simulink model "reduced_orig"  (R2018a)
settings: Solver=VariableStepAuto  StartTime=0.0  StopTime=10.0  RelTol=1e-3
undefined symbols (not defined in the file or in its folder): DiscIntNeverNeededParam
libraries: simulink x24
settings Model: Creator=ishaf  LastModifiedBy=ishaf

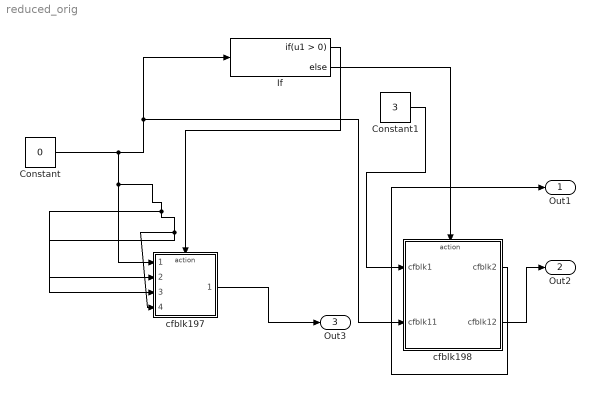
== system reduced_orig ==
  Constant : Constant  Value=0
  Constant1 : Constant  Value=3
  If : If
  cfblk197 : Subsystem  TreatAsAtomicUnit=on
  cfblk198 : Subsystem  TreatAsAtomicUnit=on
  Out1 : Outport
  Out2 : Outport  Port=2
  Out3 : Outport  Port=3
  wires:
  If/2 -> cfblk198/Action
  cfblk198/1(cfblk2) -> Out1/1
  If/1 -> cfblk197/Action
  cfblk198/2(cfblk12) -> Out2/1
  cfblk197/1(cfblk2) -> Out3/1
  Constant/1 -> cfblk197/1(cfblk1), cfblk197/2(cfblk14), cfblk197/4(cfblk16), cfblk197/3(cfblk15), cfblk198/2(cfblk11), If/1
  Constant1/1 -> cfblk198/1(cfblk1)

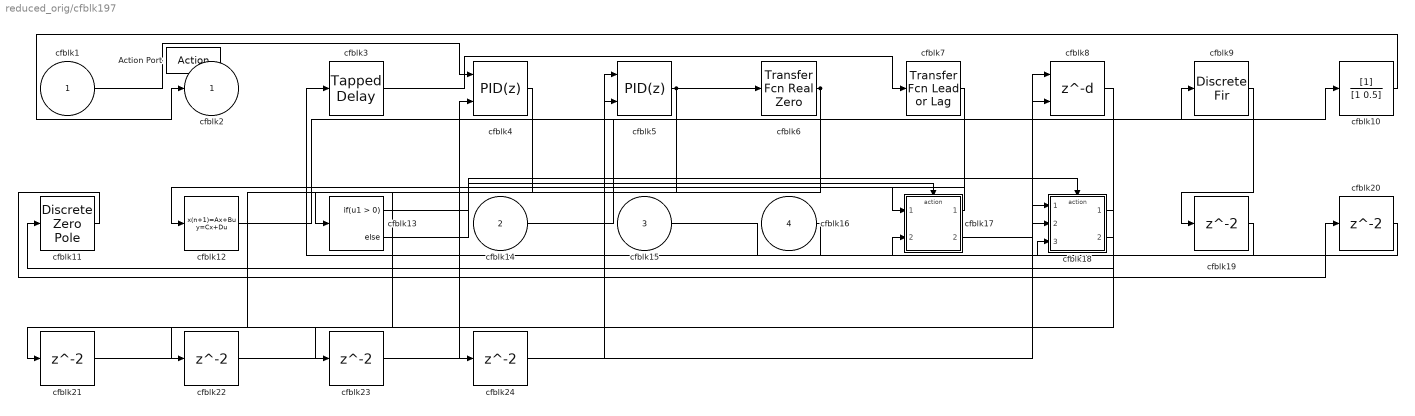
== system reduced_orig/cfblk197 ==
  cfblk1 : Inport
  cfblk14 : Inport  Port=2
  cfblk15 : Inport  Port=3
  cfblk16 : Inport  Port=4
  Action Port : ActionPort  ActionType=then
  cfblk10 : DiscreteFilter
  cfblk11 : DiscreteZeroPole  Poles=[0 0.5]  Gain=1  SampleTime=-1
  cfblk12 : DiscreteStateSpace  SampleTime=-1
  cfblk13 : If  SampleTime=1
  cfblk17 : Subsystem  TreatAsAtomicUnit=on
  cfblk18 : Subsystem  TreatAsAtomicUnit=on
  cfblk{19..24} (6 alike) : Delay
  cfblk3 : simulink/Discrete/Tapped Delay  vinit=0.0  samptime=-1  NumDelays=1  DelayOrder=Oldest  includeCurrent=off
  cfblk4 : simulink/Continuous/PID Controller (2DOF)  Controller=PID  TimeDomain=Discrete-time  SampleTime=-1  IntegratorMethod=Forward Euler  FilterMethod=Forward Euler  Form=Parallel  UseFilter=on  ControllerParametersSource=internal  P=1  I=1  D=0  N=100  b=1  c=1  InitialConditionSource=internal  InitialConditionForIntegrator=0  InitialConditionForFilter=0  ExternalReset=none  LimitOutput=off  UpperSaturationLimit=inf  LowerSaturationLimit=-inf  LinearizeAsGain=off  AntiWindupMode=none  Kb=1  TrackingMode=off  Kt=1  PParamMin=[]  PParamMax=[]  IParamMin=[]  IParamMax=[]  DParamMin=[]  DParamMax=[]  NParamMin=[]  NParamMax=[]  bParamMin=[]  bParamMax=[]  cParamMin=[]  cParamMax=[]  KbParamMin=[]  KbParamMax=[]  KtParamMin=[]  KtParamMax=[]  POutMin=[]  POutMax=[]  IOutMin=[]  IOutMax=[]  DOutMin=[]  DOutMax=[]  NOutMin=[]  NOutMax=[]  bOutMin=[]  bOutMax=[]  cOutMin=[]  cOutMax=[]  KbOutMin=[]  KbOutMax=[]  KtOutMin=[]  KtOutMax=[]  IntegratorOutMin=[]  IntegratorOutMax=[]  FilterOutMin=[]  FilterOutMax=[]  SumOutMin=[]  SumOutMax=[]  Sum1OutMin=[]  Sum1OutMax=[]  Sum2OutMin=[]  Sum2OutMax=[]  Sum3OutMin=[]  Sum3OutMax=[]  SumI1OutMin=[]  SumI1OutMax=[]  SumI2OutMin=[]  SumI2OutMax=[]  SumI3OutMin=[]  SumI3OutMax=[]  SumDOutMin=[]  SumDOutMax=[]  SaturationOutMin=[]  SaturationOutMax=[]  IntegratorContinuousStateAttributes=''  IntegratorStateMustResolveToSignalObject=off  IntegratorRTWStateStorageClass=Auto  FilterContinuousStateAttributes=''  FilterStateMustResolveToSignalObject=off  FilterRTWStateStorageClass=Auto  DifferentiatorICPrevScaledInput=0  DifferentiatorOutMin=[]  DifferentiatorOutMax=[]  FilterDiffOutCoefMin=[]  FilterDiffOutCoefMax=[]  SumDenOutMin=[]  SumDenOutMax=[]  SumNumOutMin=[]  SumNumOutMax=[]  ReciprocalOutMin=[]  ReciprocalOutMax=[]  DivideOutMin=[]  DivideOutMax=[]  TunerSelectOption=Transfer Function Based (PID Tuner App)
  cfblk5 : simulink/Continuous/PID Controller (2DOF)  Controller=PID  TimeDomain=Discrete-time  SampleTime=-1  IntegratorMethod=Forward Euler  FilterMethod=Forward Euler  Form=Parallel  UseFilter=on  ControllerParametersSource=internal  P=1  I=1  D=0  N=100  b=1  c=1  InitialConditionSource=internal  InitialConditionForIntegrator=0  InitialConditionForFilter=0  ExternalReset=none  LimitOutput=off  UpperSaturationLimit=inf  LowerSaturationLimit=-inf  LinearizeAsGain=off  AntiWindupMode=none  Kb=1  TrackingMode=off  Kt=1  PParamMin=[]  PParamMax=[]  IParamMin=[]  IParamMax=[]  DParamMin=[]  DParamMax=[]  NParamMin=[]  NParamMax=[]  bParamMin=[]  bParamMax=[]  cParamMin=[]  cParamMax=[]  KbParamMin=[]  KbParamMax=[]  KtParamMin=[]  KtParamMax=[]  POutMin=[]  POutMax=[]  IOutMin=[]  IOutMax=[]  DOutMin=[]  DOutMax=[]  NOutMin=[]  NOutMax=[]  bOutMin=[]  bOutMax=[]  cOutMin=[]  cOutMax=[]  KbOutMin=[]  KbOutMax=[]  KtOutMin=[]  KtOutMax=[]  IntegratorOutMin=[]  IntegratorOutMax=[]  FilterOutMin=[]  FilterOutMax=[]  SumOutMin=[]  SumOutMax=[]  Sum1OutMin=[]  Sum1OutMax=[]  Sum2OutMin=[]  Sum2OutMax=[]  Sum3OutMin=[]  Sum3OutMax=[]  SumI1OutMin=[]  SumI1OutMax=[]  SumI2OutMin=[]  SumI2OutMax=[]  SumI3OutMin=[]  SumI3OutMax=[]  SumDOutMin=[]  SumDOutMax=[]  SaturationOutMin=[]  SaturationOutMax=[]  IntegratorContinuousStateAttributes=''  IntegratorStateMustResolveToSignalObject=off  IntegratorRTWStateStorageClass=Auto  FilterContinuousStateAttributes=''  FilterStateMustResolveToSignalObject=off  FilterRTWStateStorageClass=Auto  DifferentiatorICPrevScaledInput=0  DifferentiatorOutMin=[]  DifferentiatorOutMax=[]  FilterDiffOutCoefMin=[]  FilterDiffOutCoefMax=[]  SumDenOutMin=[]  SumDenOutMax=[]  SumNumOutMin=[]  SumNumOutMax=[]  ReciprocalOutMin=[]  ReciprocalOutMax=[]  DivideOutMin=[]  DivideOutMax=[]  TunerSelectOption=Transfer Function Based (PID Tuner App)
  cfblk6 : simulink/Discrete/Transfer Fcn Real Zero  ZeroZ=0.75  ICPrevInput=0.0  DoSatur=off
      settings: SourceProductName=Simulink  SourceProductBaseCode=SL
  cfblk7 : simulink/Discrete/Transfer Fcn Lead or Lag  PoleZ=0.95  ZeroZ=0.75  ICPrevOutput=0.0  ICPrevInput=0.0  DoSatur=off
      settings: SourceProductName=Simulink  SourceProductBaseCode=SL
  cfblk8 : Delay  DelayLengthSource=Input port
      settings: InputPortMap=u0,p1
  cfblk9 : DiscreteFir
  cfblk2 : Outport
  wires:
  cfblk3/1 -> cfblk7/1
  cfblk5/1 -> cfblk6/1, cfblk22/1
  cfblk1/1 -> cfblk4/1
  cfblk4/1 -> cfblk13/1
  cfblk16/1 -> cfblk3/1
  cfblk8/1 -> cfblk11/1
  cfblk15/1 -> cfblk18/3(cfblk10)
  cfblk6/1 -> cfblk23/1, cfblk24/1
  cfblk10/1 -> cfblk2/1
  cfblk7/1 -> cfblk17/1(cfblk1)
  cfblk14/1 -> cfblk10/1
  cfblk12/1 -> cfblk9/1
  cfblk17/1(cfblk2) -> cfblk12/1
  cfblk17/2(cfblk17) -> cfblk8/2
  cfblk18/2(cfblk11) -> cfblk5/1
  cfblk13/1 -> cfblk17/Action
  cfblk13/2 -> cfblk18/Action
  cfblk9/1 -> cfblk19/1
  cfblk19/1 -> cfblk17/2(cfblk16)
  cfblk11/1 -> cfblk20/1
  cfblk20/1 -> cfblk18/2(cfblk9)
  cfblk18/1(cfblk2) -> cfblk21/1
  cfblk21/1 -> cfblk4/2
  cfblk22/1 -> cfblk18/1(cfblk1)
  cfblk23/1 -> cfblk8/1
  cfblk24/1 -> cfblk5/2

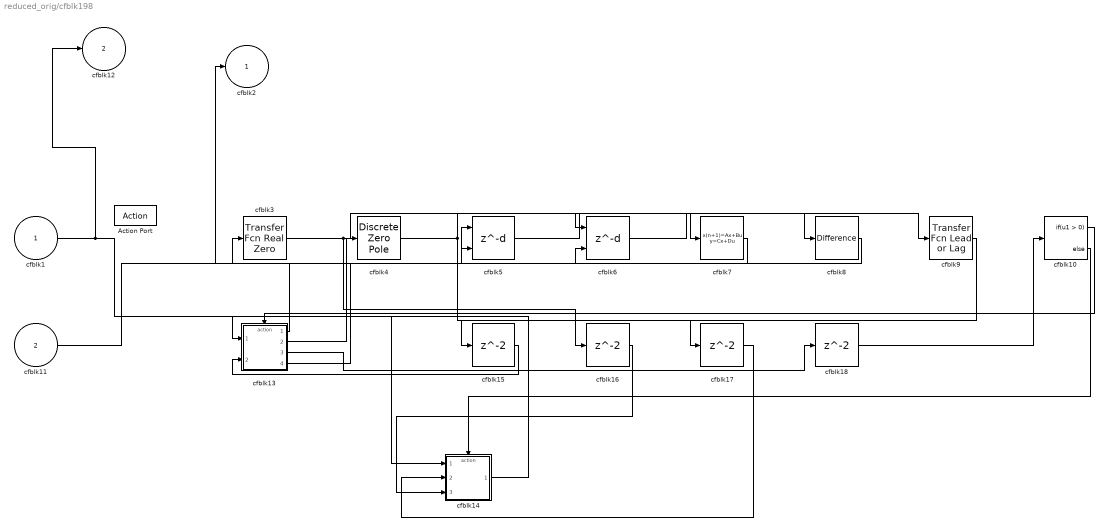
== system reduced_orig/cfblk198 ==
  cfblk1 : Inport
  cfblk11 : Inport  Port=2
  Action Port : ActionPort  ActionType=else
  cfblk10 : If  SampleTime=1
  cfblk13 : Subsystem  TreatAsAtomicUnit=on
  cfblk14 : Subsystem  TreatAsAtomicUnit=on
  cfblk{15..18} (4 alike) : Delay
  cfblk3 : simulink/Discrete/Transfer Fcn Real Zero  ZeroZ=0.75  ICPrevInput=0.0  DoSatur=off
      settings: SourceProductName=Simulink  SourceProductBaseCode=SL
  cfblk4 : DiscreteZeroPole  Poles=[0 0.5]  Gain=1  SampleTime=-1
  cfblk5 : Delay  DelayLengthSource=Input port
      settings: InputPortMap=u0,p1
  cfblk6 : Delay  DelayLengthSource=Input port
      settings: InputPortMap=u0,p1
  cfblk7 : DiscreteStateSpace  SampleTime=-1
  cfblk8 : simulink/Discrete/Difference  ICPrevInput=0.0  OutMin=[]  OutMax=[]  OutDataTypeStr=Inherit: Inherit via back propagation  OutDataType=fixdt(1, 16)  OutScaling=2^-10  DoSatur=off
  cfblk9 : simulink/Discrete/Transfer Fcn Lead or Lag  PoleZ=0.95  ZeroZ=0.75  ICPrevOutput=0.0  ICPrevInput=0.0  DoSatur=off
      settings: SourceProductName=Simulink  SourceProductBaseCode=SL
  cfblk2 : Outport
  cfblk12 : Outport  Port=2
  wires:
  cfblk5/1 -> cfblk9/1
  cfblk8/1 -> cfblk5/1
  cfblk3/1 -> cfblk6/1, cfblk16/1
  cfblk14/1(cfblk2) -> cfblk13/1(cfblk1)
  cfblk7/1 -> cfblk2/1
  cfblk11/1 -> cfblk5/2
  cfblk1/1 -> cfblk12/1, cfblk14/1(cfblk1)
  cfblk4/1 -> cfblk7/1, cfblk17/1
  cfblk6/1 -> cfblk8/1
  cfblk13/1(cfblk2) -> cfblk3/1
  cfblk13/2(cfblk14) -> cfblk4/1
  cfblk13/4(cfblk16) -> cfblk6/2
  cfblk10/1 -> cfblk13/Action
  cfblk10/2 -> cfblk14/Action
  cfblk9/1 -> cfblk15/1
  cfblk15/1 -> cfblk13/2(cfblk13)
  cfblk16/1 -> cfblk14/3(cfblk12)
  cfblk17/1 -> cfblk14/2(cfblk11)
  cfblk13/3(cfblk15) -> cfblk18/1
  cfblk18/1 -> cfblk10/1

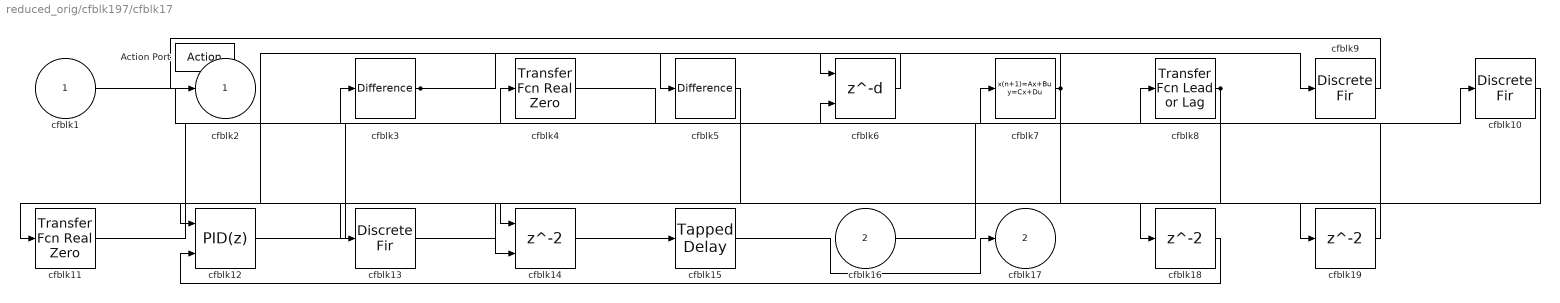
== system reduced_orig/cfblk197/cfblk17 ==
  cfblk1 : Inport
  cfblk16 : Inport  Port=2
  Action Port : ActionPort  ActionType=then
  cfblk10 : DiscreteFir
  cfblk11 : simulink/Discrete/Transfer Fcn Real Zero  ZeroZ=0.75  ICPrevInput=0.0  DoSatur=off
      settings: SourceProductName=Simulink  SourceProductBaseCode=SL
  cfblk12 : simulink/Continuous/PID Controller (2DOF)  Controller=PID  TimeDomain=Discrete-time  SampleTime=-1  IntegratorMethod=Forward Euler  FilterMethod=Forward Euler  Form=Parallel  UseFilter=on  ControllerParametersSource=internal  P=1  I=1  D=0  N=100  b=1  c=1  InitialConditionSource=internal  InitialConditionForIntegrator=0  InitialConditionForFilter=0  ExternalReset=none  LimitOutput=off  UpperSaturationLimit=inf  LowerSaturationLimit=-inf  LinearizeAsGain=off  AntiWindupMode=none  Kb=1  TrackingMode=off  Kt=1  PParamMin=[]  PParamMax=[]  IParamMin=[]  IParamMax=[]  DParamMin=[]  DParamMax=[]  NParamMin=[]  NParamMax=[]  bParamMin=[]  bParamMax=[]  cParamMin=[]  cParamMax=[]  KbParamMin=[]  KbParamMax=[]  KtParamMin=[]  KtParamMax=[]  POutMin=[]  POutMax=[]  IOutMin=[]  IOutMax=[]  DOutMin=[]  DOutMax=[]  NOutMin=[]  NOutMax=[]  bOutMin=[]  bOutMax=[]  cOutMin=[]  cOutMax=[]  KbOutMin=[]  KbOutMax=[]  KtOutMin=[]  KtOutMax=[]  IntegratorOutMin=[]  IntegratorOutMax=[]  FilterOutMin=[]  FilterOutMax=[]  SumOutMin=[]  SumOutMax=[]  Sum1OutMin=[]  Sum1OutMax=[]  Sum2OutMin=[]  Sum2OutMax=[]  Sum3OutMin=[]  Sum3OutMax=[]  SumI1OutMin=[]  SumI1OutMax=[]  SumI2OutMin=[]  SumI2OutMax=[]  SumI3OutMin=[]  SumI3OutMax=[]  SumDOutMin=[]  SumDOutMax=[]  SaturationOutMin=[]  SaturationOutMax=[]  IntegratorContinuousStateAttributes=''  IntegratorStateMustResolveToSignalObject=off  IntegratorRTWStateStorageClass=Auto  FilterContinuousStateAttributes=''  FilterStateMustResolveToSignalObject=off  FilterRTWStateStorageClass=Auto  DifferentiatorICPrevScaledInput=0  DifferentiatorOutMin=[]  DifferentiatorOutMax=[]  FilterDiffOutCoefMin=[]  FilterDiffOutCoefMax=[]  SumDenOutMin=[]  SumDenOutMax=[]  SumNumOutMin=[]  SumNumOutMax=[]  ReciprocalOutMin=[]  ReciprocalOutMax=[]  DivideOutMin=[]  DivideOutMax=[]  TunerSelectOption=Transfer Function Based (PID Tuner App)
  cfblk13 : DiscreteFir
  cfblk14 : Delay  ShowEnablePort=on
      settings: InputPortMap=u0,e6
  cfblk15 : simulink/Discrete/Tapped Delay  vinit=0.0  samptime=-1  NumDelays=1  DelayOrder=Oldest  includeCurrent=off
  cfblk18 : Delay
  cfblk19 : Delay
  cfblk3 : simulink/Discrete/Difference  ICPrevInput=0.0  OutMin=[]  OutMax=[]  OutDataTypeStr=Inherit: Inherit via back propagation  OutDataType=fixdt(1, 16)  OutScaling=2^-10  DoSatur=off
  cfblk4 : simulink/Discrete/Transfer Fcn Real Zero  ZeroZ=0.75  ICPrevInput=0.0  DoSatur=off
      settings: SourceProductName=Simulink  SourceProductBaseCode=SL
  cfblk5 : simulink/Discrete/Difference  ICPrevInput=0.0  OutMin=[]  OutMax=[]  OutDataTypeStr=Inherit: Inherit via back propagation  OutDataType=fixdt(1, 16)  OutScaling=2^-10  DoSatur=off
  cfblk6 : Delay  DelayLengthSource=Input port
      settings: InputPortMap=u0,p1
  cfblk7 : DiscreteStateSpace  SampleTime=-1
  cfblk8 : simulink/Discrete/Transfer Fcn Lead or Lag  PoleZ=0.95  ZeroZ=0.75  ICPrevOutput=0.0  ICPrevInput=0.0  DoSatur=off
      settings: SourceProductName=Simulink  SourceProductBaseCode=SL
  cfblk9 : DiscreteFir
  cfblk2 : Outport
  cfblk17 : Outport  Port=2
  wires:
  cfblk14/1 -> cfblk15/1
  cfblk10/1 -> cfblk14/1
  cfblk12/1 -> cfblk8/1
  cfblk15/1 -> cfblk17/1
  cfblk7/1 -> cfblk11/1, cfblk13/1
  cfblk6/1 -> cfblk5/1
  cfblk9/1 -> cfblk2/1
  cfblk11/1 -> cfblk3/1
  cfblk1/1 -> cfblk4/1
  cfblk3/1 -> cfblk6/1, cfblk9/1
  cfblk5/1 -> cfblk12/1
  cfblk16/1 -> cfblk10/1
  cfblk8/1 -> cfblk14/2, cfblk18/1
  cfblk4/1 -> cfblk6/2
  cfblk18/1 -> cfblk12/2
  cfblk13/1 -> cfblk19/1
  cfblk19/1 -> cfblk7/1

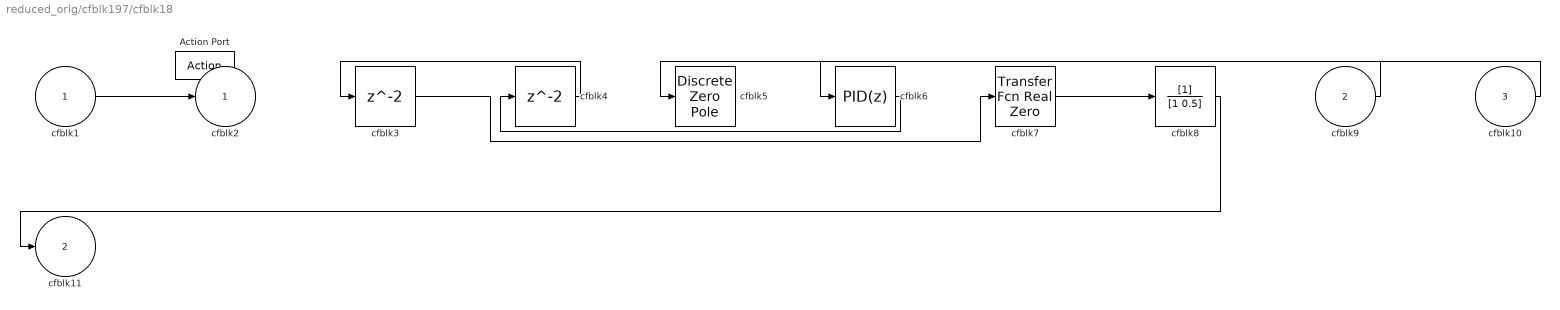
== system reduced_orig/cfblk197/cfblk18 ==
  cfblk1 : Inport
  cfblk9 : Inport  Port=2
  cfblk10 : Inport  Port=3
  Action Port : ActionPort  ActionType=else
  cfblk3 : Delay
  cfblk4 : Delay
  cfblk5 : DiscreteZeroPole  Poles=[0 0.5]  Gain=1  SampleTime=-1
  cfblk6 : simulink/Continuous/PID Controller  Controller=PID  TimeDomain=Discrete-time  SampleTime=-1  IntegratorMethod=Forward Euler  FilterMethod=Forward Euler  Form=Parallel  UseFilter=on  ControllerParametersSource=internal  P=1  I=1  D=0  N=100  InitialConditionSource=internal  InitialConditionForIntegrator=0  InitialConditionForFilter=0  ExternalReset=none  LimitOutput=off  UpperSaturationLimit=inf  LowerSaturationLimit=-inf  LinearizeAsGain=off  AntiWindupMode=none  Kb=1  TrackingMode=off  Kt=1  PParamMin=[]  PParamMax=[]  IParamMin=[]  IParamMax=[]  DParamMin=[]  DParamMax=[]  NParamMin=[]  NParamMax=[]  KbParamMin=[]  KbParamMax=[]  KtParamMin=[]  KtParamMax=[]  POutMin=[]  POutMax=[]  IOutMin=[]  IOutMax=[]  DOutMin=[]  DOutMax=[]  NOutMin=[]  NOutMax=[]  KbOutMin=[]  KbOutMax=[]  KtOutMin=[]  KtOutMax=[]  IntegratorOutMin=[]  IntegratorOutMax=[]  FilterOutMin=[]  FilterOutMax=[]  SumOutMin=[]  SumOutMax=[]  SumI1OutMin=[]  SumI1OutMax=[]  SumI2OutMin=[]  SumI2OutMax=[]  SumI3OutMin=[]  SumI3OutMax=[]  SumDOutMin=[]  SumDOutMax=[]  SaturationOutMin=[]  SaturationOutMax=[]  IntegratorContinuousStateAttributes=''  IntegratorStateMustResolveToSignalObject=off  IntegratorRTWStateStorageClass=Auto  FilterContinuousStateAttributes=''  FilterStateMustResolveToSignalObject=off  FilterRTWStateStorageClass=Auto  DifferentiatorICPrevScaledInput=0  DifferentiatorOutMin=[]  DifferentiatorOutMax=[]  FilterDiffOutCoefMin=[]  FilterDiffOutCoefMax=[]  SumDenOutMin=[]  SumDenOutMax=[]  SumNumOutMin=[]  SumNumOutMax=[]  ReciprocalOutMin=[]  ReciprocalOutMax=[]  DivideOutMin=[]  DivideOutMax=[]  TunerSelectOption=Transfer Function Based (PID Tuner App)
  cfblk7 : simulink/Discrete/Transfer Fcn Real Zero  ZeroZ=0.75  ICPrevInput=0.0  DoSatur=off
      settings: SourceProductName=Simulink  SourceProductBaseCode=SL
  cfblk8 : DiscreteFilter
  cfblk2 : Outport
  cfblk11 : Outport  Port=2
  wires:
  cfblk10/1 -> cfblk6/1
  cfblk6/1 -> cfblk4/1
  cfblk7/1 -> cfblk8/1
  cfblk8/1 -> cfblk11/1
  cfblk1/1 -> cfblk2/1
  cfblk3/1 -> cfblk7/1
  cfblk4/1 -> cfblk3/1
  cfblk9/1 -> cfblk5/1

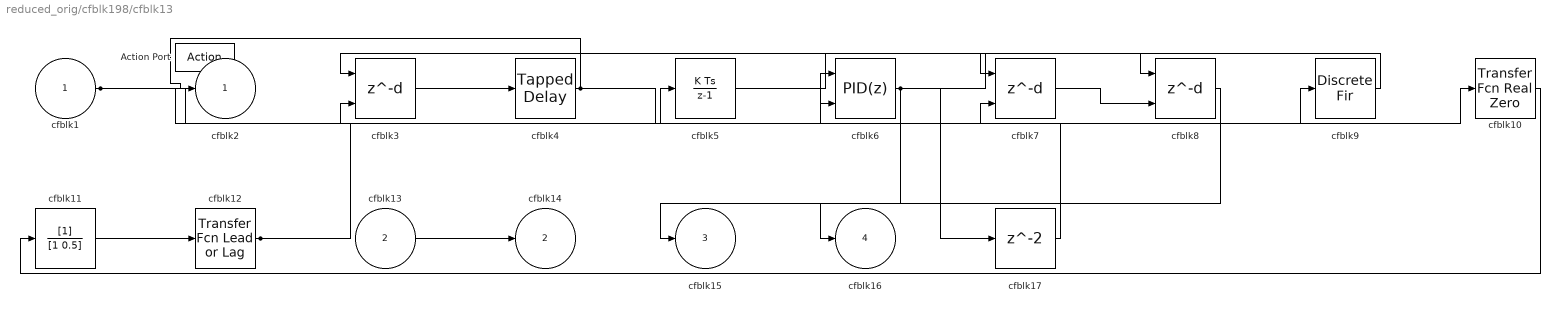
== system reduced_orig/cfblk198/cfblk13 ==
  cfblk1 : Inport
  cfblk13 : Inport  Port=2
  Action Port : ActionPort  ActionType=then
  cfblk10 : simulink/Discrete/Transfer Fcn Real Zero  ZeroZ=0.75  ICPrevInput=0.0  DoSatur=off
      settings: SourceProductName=Simulink  SourceProductBaseCode=SL
  cfblk11 : DiscreteFilter
  cfblk12 : simulink/Discrete/Transfer Fcn Lead or Lag  PoleZ=0.95  ZeroZ=0.75  ICPrevOutput=0.0  ICPrevInput=0.0  DoSatur=off
      settings: SourceProductName=Simulink  SourceProductBaseCode=SL
  cfblk17 : Delay
  cfblk3 : Delay  DelayLengthSource=Input port
      settings: InputPortMap=u0,p1
  cfblk4 : simulink/Discrete/Tapped Delay  vinit=0.0  samptime=-1  NumDelays=1  DelayOrder=Oldest  includeCurrent=off
  cfblk5 : DiscreteIntegrator  SampleTime=-1  ICPrevOutput=DiscIntNeverNeededParam  ICPrevScaledInput=DiscIntNeverNeededParam
  cfblk6 : simulink/Continuous/PID Controller (2DOF)  Controller=PID  TimeDomain=Discrete-time  SampleTime=-1  IntegratorMethod=Forward Euler  FilterMethod=Forward Euler  Form=Parallel  UseFilter=on  ControllerParametersSource=internal  P=1  I=1  D=0  N=100  b=1  c=1  InitialConditionSource=internal  InitialConditionForIntegrator=0  InitialConditionForFilter=0  ExternalReset=none  LimitOutput=off  UpperSaturationLimit=inf  LowerSaturationLimit=-inf  LinearizeAsGain=off  AntiWindupMode=none  Kb=1  TrackingMode=off  Kt=1  PParamMin=[]  PParamMax=[]  IParamMin=[]  IParamMax=[]  DParamMin=[]  DParamMax=[]  NParamMin=[]  NParamMax=[]  bParamMin=[]  bParamMax=[]  cParamMin=[]  cParamMax=[]  KbParamMin=[]  KbParamMax=[]  KtParamMin=[]  KtParamMax=[]  POutMin=[]  POutMax=[]  IOutMin=[]  IOutMax=[]  DOutMin=[]  DOutMax=[]  NOutMin=[]  NOutMax=[]  bOutMin=[]  bOutMax=[]  cOutMin=[]  cOutMax=[]  KbOutMin=[]  KbOutMax=[]  KtOutMin=[]  KtOutMax=[]  IntegratorOutMin=[]  IntegratorOutMax=[]  FilterOutMin=[]  FilterOutMax=[]  SumOutMin=[]  SumOutMax=[]  Sum1OutMin=[]  Sum1OutMax=[]  Sum2OutMin=[]  Sum2OutMax=[]  Sum3OutMin=[]  Sum3OutMax=[]  SumI1OutMin=[]  SumI1OutMax=[]  SumI2OutMin=[]  SumI2OutMax=[]  SumI3OutMin=[]  SumI3OutMax=[]  SumDOutMin=[]  SumDOutMax=[]  SaturationOutMin=[]  SaturationOutMax=[]  IntegratorContinuousStateAttributes=''  IntegratorStateMustResolveToSignalObject=off  IntegratorRTWStateStorageClass=Auto  FilterContinuousStateAttributes=''  FilterStateMustResolveToSignalObject=off  FilterRTWStateStorageClass=Auto  DifferentiatorICPrevScaledInput=0  DifferentiatorOutMin=[]  DifferentiatorOutMax=[]  FilterDiffOutCoefMin=[]  FilterDiffOutCoefMax=[]  SumDenOutMin=[]  SumDenOutMax=[]  SumNumOutMin=[]  SumNumOutMax=[]  ReciprocalOutMin=[]  ReciprocalOutMax=[]  DivideOutMin=[]  DivideOutMax=[]  TunerSelectOption=Transfer Function Based (PID Tuner App)
  cfblk7 : Delay  DelayLengthSource=Input port
      settings: InputPortMap=u0,p1
  cfblk8 : Delay  DelayLengthSource=Input port
      settings: InputPortMap=u0,p1
  cfblk9 : DiscreteFir
  cfblk2 : Outport
  cfblk14 : Outport  Port=2
  cfblk15 : Outport  Port=3
  cfblk16 : Outport  Port=4
  wires:
  cfblk11/1 -> cfblk12/1
  cfblk1/1 -> cfblk10/1, cfblk7/2, cfblk6/1
  cfblk4/1 -> cfblk2/1, cfblk6/2
  cfblk12/1 -> cfblk5/1, cfblk9/1
  cfblk13/1 -> cfblk14/1
  cfblk6/1 -> cfblk8/1, cfblk15/1, cfblk17/1
  cfblk9/1 -> cfblk3/1
  cfblk10/1 -> cfblk11/1
  cfblk3/1 -> cfblk4/1
  cfblk5/1 -> cfblk7/1
  cfblk7/1 -> cfblk8/2
  cfblk8/1 -> cfblk16/1
  cfblk17/1 -> cfblk3/2

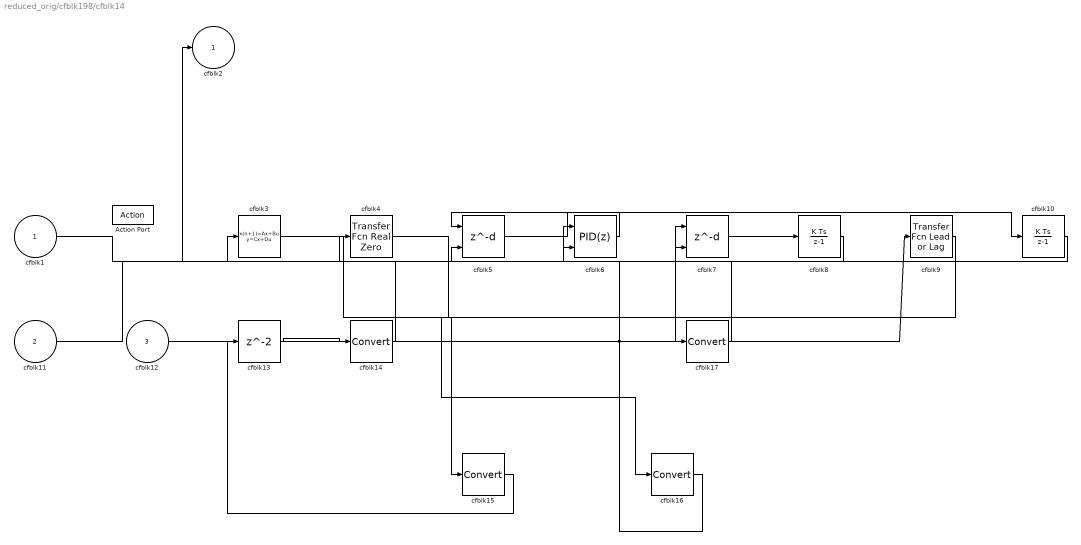
== system reduced_orig/cfblk198/cfblk14 ==
  cfblk1 : Inport
  cfblk11 : Inport  Port=2
  cfblk12 : Inport  Port=3
  Action Port : ActionPort  ActionType=else
  cfblk10 : DiscreteIntegrator  SampleTime=-1  ICPrevOutput=DiscIntNeverNeededParam  ICPrevScaledInput=DiscIntNeverNeededParam
  cfblk13 : Delay
  cfblk{14..17} (4 alike) : DataTypeConversion
  cfblk3 : DiscreteStateSpace  SampleTime=-1
  cfblk4 : simulink/Discrete/Transfer Fcn Real Zero  ZeroZ=0.75  ICPrevInput=0.0  DoSatur=off
      settings: SourceProductName=Simulink  SourceProductBaseCode=SL
  cfblk5 : Delay  DelayLengthSource=Input port
      settings: InputPortMap=u0,p1
  cfblk6 : simulink/Continuous/PID Controller (2DOF)  Controller=PID  TimeDomain=Discrete-time  SampleTime=-1  IntegratorMethod=Forward Euler  FilterMethod=Forward Euler  Form=Parallel  UseFilter=on  ControllerParametersSource=internal  P=1  I=1  D=0  N=100  b=1  c=1  InitialConditionSource=internal  InitialConditionForIntegrator=0  InitialConditionForFilter=0  ExternalReset=none  LimitOutput=off  UpperSaturationLimit=inf  LowerSaturationLimit=-inf  LinearizeAsGain=off  AntiWindupMode=none  Kb=1  TrackingMode=off  Kt=1  PParamMin=[]  PParamMax=[]  IParamMin=[]  IParamMax=[]  DParamMin=[]  DParamMax=[]  NParamMin=[]  NParamMax=[]  bParamMin=[]  bParamMax=[]  cParamMin=[]  cParamMax=[]  KbParamMin=[]  KbParamMax=[]  KtParamMin=[]  KtParamMax=[]  POutMin=[]  POutMax=[]  IOutMin=[]  IOutMax=[]  DOutMin=[]  DOutMax=[]  NOutMin=[]  NOutMax=[]  bOutMin=[]  bOutMax=[]  cOutMin=[]  cOutMax=[]  KbOutMin=[]  KbOutMax=[]  KtOutMin=[]  KtOutMax=[]  IntegratorOutMin=[]  IntegratorOutMax=[]  FilterOutMin=[]  FilterOutMax=[]  SumOutMin=[]  SumOutMax=[]  Sum1OutMin=[]  Sum1OutMax=[]  Sum2OutMin=[]  Sum2OutMax=[]  Sum3OutMin=[]  Sum3OutMax=[]  SumI1OutMin=[]  SumI1OutMax=[]  SumI2OutMin=[]  SumI2OutMax=[]  SumI3OutMin=[]  SumI3OutMax=[]  SumDOutMin=[]  SumDOutMax=[]  SaturationOutMin=[]  SaturationOutMax=[]  IntegratorContinuousStateAttributes=''  IntegratorStateMustResolveToSignalObject=off  IntegratorRTWStateStorageClass=Auto  FilterContinuousStateAttributes=''  FilterStateMustResolveToSignalObject=off  FilterRTWStateStorageClass=Auto  DifferentiatorICPrevScaledInput=0  DifferentiatorOutMin=[]  DifferentiatorOutMax=[]  FilterDiffOutCoefMin=[]  FilterDiffOutCoefMax=[]  SumDenOutMin=[]  SumDenOutMax=[]  SumNumOutMin=[]  SumNumOutMax=[]  ReciprocalOutMin=[]  ReciprocalOutMax=[]  DivideOutMin=[]  DivideOutMax=[]  TunerSelectOption=Transfer Function Based (PID Tuner App)
  cfblk7 : Delay  DelayLengthSource=Input port
      settings: InputPortMap=u0,p1
  cfblk8 : DiscreteIntegrator  SampleTime=-1  ICPrevOutput=DiscIntNeverNeededParam  ICPrevScaledInput=DiscIntNeverNeededParam
  cfblk9 : simulink/Discrete/Transfer Fcn Lead or Lag  PoleZ=0.95  ZeroZ=0.75  ICPrevOutput=0.0  ICPrevInput=0.0  DoSatur=off
      settings: SourceProductName=Simulink  SourceProductBaseCode=SL
  cfblk2 : Outport
  wires:
  cfblk5/1 -> cfblk10/1
  cfblk7/1 -> cfblk8/1
  cfblk10/1 -> cfblk2/1
  cfblk11/1 -> cfblk7/1
  cfblk4/1 -> cfblk16/1
  cfblk12/1 -> cfblk7/2
  cfblk1/1 -> cfblk6/1
  cfblk8/1 -> cfblk6/2
  cfblk6/1 -> cfblk5/1
  cfblk13/1 -> cfblk14/1
  cfblk14/1 -> cfblk3/1
  cfblk9/1 -> cfblk15/1
  cfblk15/1 -> cfblk13/1
  cfblk16/1 -> cfblk5/2, cfblk9/1
  cfblk3/1 -> cfblk17/1
  cfblk17/1 -> cfblk4/1
